simulink model "GUI_simulink"  (R2024b)
settings: Solver=ode45  StartTime=0.0  StopTime=15.0  MaxStep=0.02  MinStep=0.01  RelTol=1e-3
settings Model: Creator=lw53894  LastModifiedBy=lw53894
settings SolverCC: InitialStep=0.01

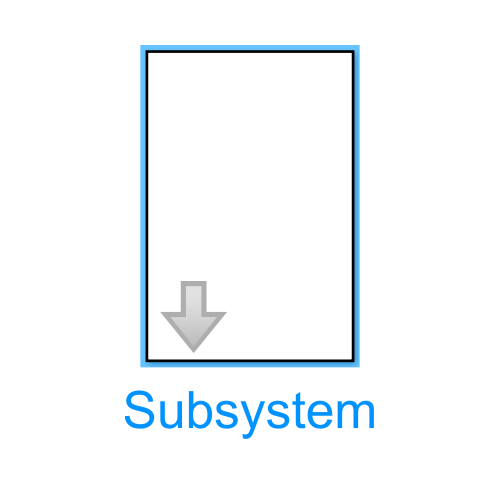
[thumbnail: Simulink's stored preview of the top-level diagram]
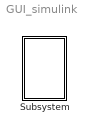
== system GUI_simulink ==
  Subsystem : Subsystem  mask{n=3, g=9.81, k=1, m=2, l=4, x=-1, y=-1, xi=[-1 1 1], yi=[1 1 -1], di=[0.1 0.1 0.1], ai=[1 -1 1.5]}

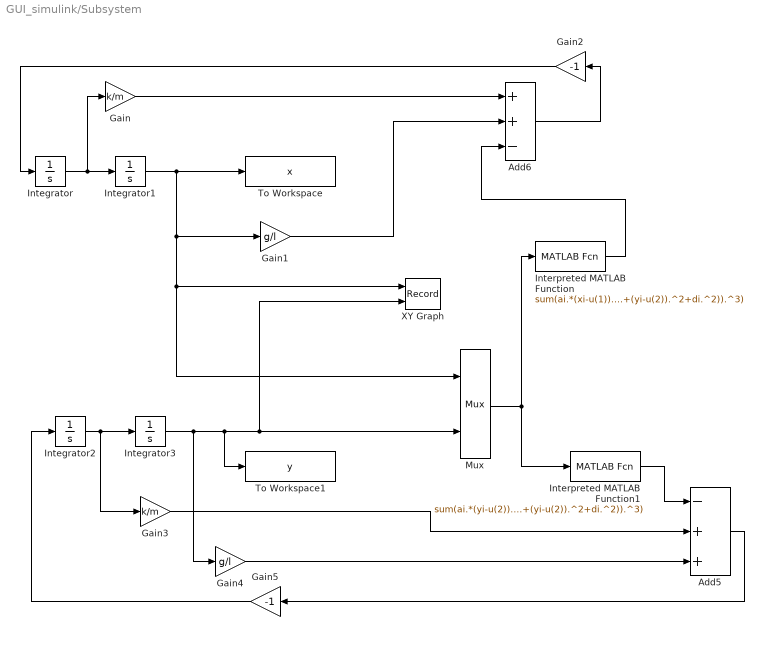
== system GUI_simulink/Subsystem ==
  Add5 : Sum  Inputs=-++
  Add6 : Sum  Inputs=++-
  Gain : Gain  Gain=k/m
  Gain1 : Gain  Gain=g/l
  Gain2 : Gain  Gain=-1
  Gain3 : Gain  Gain=k/m
  Gain4 : Gain  Gain=g/l
  Gain5 : Gain  Gain=-1
  Integrator : Integrator
  Integrator1 : Integrator  InitialCondition=x
  Integrator2 : Integrator
  Integrator3 : Integrator  InitialCondition=y
  Interpreted MATLAB Function : MATLABFcn  MATLABFcn=sum(ai.*(xi-u(1))./(sqrt((xi-u(1)).^2+(yi-u(2)).^2+di.^2)).^3)
  Interpreted MATLAB Function1 : MATLABFcn  MATLABFcn=sum(ai.*(yi-u(2))./(sqrt((xi-u(1)).^2+(yi-u(2)).^2+di.^2)).^3)
  Mux : Mux  Inputs=2
  To Workspace : ToWorkspace  VariableName=x  SaveFormat=Timeseries  SampleTime=-1
  To Workspace1 : ToWorkspace  VariableName=y  SaveFormat=Timeseries  SampleTime=-1
  XY Graph : Record  FileSettingsInternal="{\"entries\":[{\"content\":{\"excelSettings\":{\"content\":{},\"type\":\"Streamout.ExcelSettings\"}},\"type\":\"Streamout.FileSettingStorage\",\"uuid\":\"\"}],\"packageUris\":[\"http:\\/\\/schema.mathworks.com\\/mf0\\/streamout_blocks\\/R2020a\"],\"version\":\"1.0\"}"  Layout=[1 1]  SignalsInternal="{\"entries\":[{\"content\":{\"signals\":[{\"content\":{\"blockPath\":[],\"dimensions\":[1],\"domain\":\"\",\"lineColor\":\"#a2142f\",\"plots\":[ 1 ],\"port\":1,\"sid\":[\"\"],\"signalID\":1,\"signalName\":\"Integrator1\"},\"type\":\"RecordBlkView.Signal\",\"uuid\":\"\"},{\"content\":{\"blockPath\":[],\"dimensions\":[1],\"domain\":\"\",\"lineColor\":\"#139fff\",\"plots\":[ 1 ],\"port\":2,\"sid\":[\"\"],\"signalID\":2,\"signalName\":\"Integrator3\"},\"type\":\"RecordBlkView.Signal\",\"uuid\":\"\"}]},\"type\":\"RecordBlkView.InputSignals\",\"uuid\":\"\"}],\"packageUris\":[\"http:\\/\\/schema.mathworks.com\\/mf0\\/streamout_blocks\\/R2020a\"],\"version\":\"1.0\"}"  VisualizationBindings="{\"xyplotplugin\":{\"info\":[{\"series\":[{\"bindingParametersList\":[{\"parameter\":\"X-Axis\",\"signalID\":1,\"signalName\":\"Integrator1\"},{\"parameter\":\"Y-Axis\",\"signalID\":2,\"signalName\":\"Integrator3\"}],\"seriesID\":0}],\"subplotID\":1}]}}"  CompatibilityTag=XY
  wires:
  Integrator/1 -> Gain/1, Integrator1/1
  Integrator2/1 -> Gain3/1, Integrator3/1
  Integrator1/1 -> To Workspace/1, XY Graph/1, Mux/1, Gain1/1
  Integrator3/1 -> Gain4/1, To Workspace1/1, XY Graph/2, Mux/2
  Add5/1 -> Gain5/1
  Mux/1 -> Interpreted MATLAB Function1/1, Interpreted MATLAB Function/1
  Interpreted MATLAB Function1/1 -> Add5/1
  Gain2/1 -> Integrator/1
  Gain5/1 -> Integrator2/1
  Gain/1 -> Add6/1
  Gain1/1 -> Add6/2
  Interpreted MATLAB Function/1 -> Add6/3
  Add6/1 -> Gain2/1
  Gain3/1 -> Add5/2
  Gain4/1 -> Add5/3
